simulink model "Solver"  (R2020a)
settings: Solver=ode23tb  StartTime=0.0  StopTime=10  RelTol=1e-3
settings Model: Creator=Mr Mejia  LastModifiedBy=Mr Mejia
settings DataIOCC: SaveFormat=Array

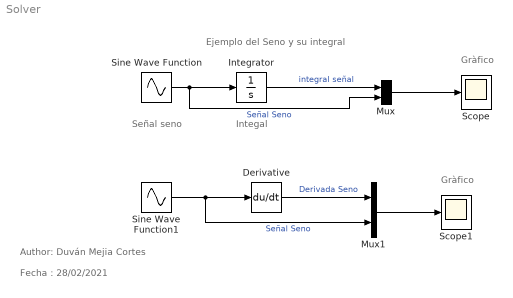
== system Solver ==
  note: Fecha : 28/02/2021
  note: Author: Duván Mejia Cortes
  note: Integal
  note: Señal seno
  note: Ejemplo del Seno y su integral
  note: Gràfico
  note: Gràfico
  Derivative : Derivative
  Integrator : Integrator
  Mux : Mux  Inputs=2
  Mux1 : Mux  Inputs=2
  Scope : Scope
  Scope1 : Scope
  Sine Wave Function : Sin  Amplitude=2  Frequency=2 * pi  Phase=pi/4  SampleTime=0
  Sine Wave Function1 : Sin  Amplitude=2  Frequency=2 * pi  Phase=pi/4  SampleTime=0
  wires:
  Sine Wave Function/1 -> Mux/2, Integrator/1  "Señal Seno"
  Integrator/1 -> Mux/1  "integral señal"
  Mux/1 -> Scope/1
  Sine Wave Function1/1 -> Mux1/2, Derivative/1  "Señal Seno"
  Derivative/1 -> Mux1/1  "Derivada Seno"
  Mux1/1 -> Scope1/1
